simulink model "TemperatureControl"  (R2023b)
settings: Solver=VariableStepAuto  StartTime=0.0  StopTime=10.0  RelTol=1e-3
model workspace (MAT data in the model file):
  COOLING = 1
  TEMPDES = 2
  agentf = 1
libraries: rllib x1
settings Model: Creator=mail  LastModifiedBy=juliu
settings DebuggingCC: UnconnectedInputMsg=warning  UnconnectedOutputMsg=warning  UnconnectedLineMsg=warning
settings ModelReferenceCC: EnableRefExpFcnMdlSchedulingChecks=on
settings RTWCC: DLArmComputeVersion=19.05

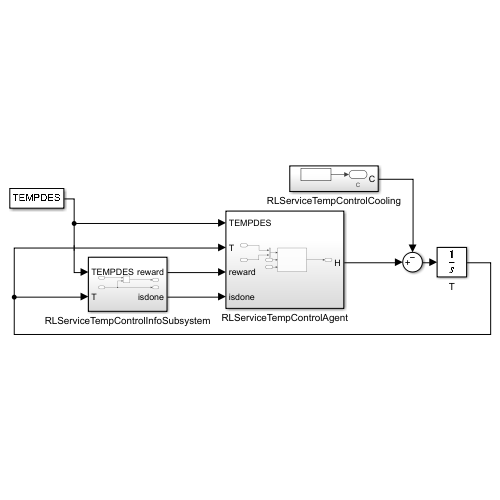
[thumbnail: Simulink's stored preview of the top-level diagram]
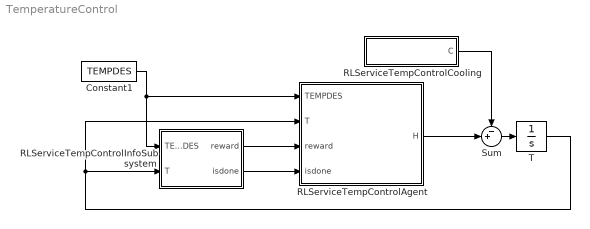
== system TemperatureControl ==
  Constant1 : Constant  Value=TEMPDES
  RLServiceTempControlAgent : Subsystem
  RLServiceTempControlCooling : Subsystem
  RLServiceTempControlInfoSubsystem : Subsystem
  Sum : Sum  Inputs=-+|
  T : Integrator
  wires:
  Sum/1 -> T/1
  T/1 -> RLServiceTempControlInfoSubsystem/2(T), RLServiceTempControlAgent/2(T)
  Constant1/1 -> RLServiceTempControlInfoSubsystem/1(TEMPDES), RLServiceTempControlAgent/1(TEMPDES)
  RLServiceTempControlInfoSubsystem/1(reward) -> RLServiceTempControlAgent/3(reward)
  RLServiceTempControlInfoSubsystem/2(isdone) -> RLServiceTempControlAgent/4(isdone)
  RLServiceTempControlAgent/1(H) -> Sum/2
  RLServiceTempControlCooling/1(C) -> Sum/1

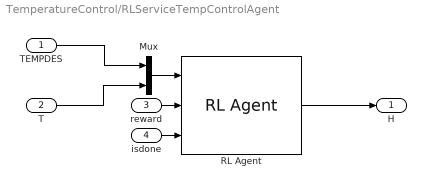
== system TemperatureControl/RLServiceTempControlAgent ==
  TEMPDES : Inport
  T : Inport  Port=2
  reward : Inport  Port=3
  isdone : Inport  Port=4
  Mux : Mux  Inputs=2
  RL Agent : rllib/RL Agent  Agent=agentf  ExternalActionAsInput=off  ProvideCumRwd=off  TreatAsDirectFeedthrough=on
  H : Outport
  wires:
  T/1 -> Mux/2
  isdone/1 -> RL Agent/3
  reward/1 -> RL Agent/2
  RL Agent/1 -> H/1
  TEMPDES/1 -> Mux/1
  Mux/1 -> RL Agent/1

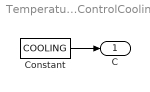
== system TemperatureControl/RLServiceTempControlCooling ==
  Constant : Constant  Value=COOLING
  C : Outport
  wires:
  Constant/1 -> C/1

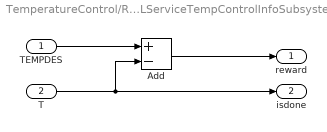
== system TemperatureControl/RLServiceTempControlInfoSubsystem ==
  TEMPDES : Inport
  T : Inport  Port=2
  Add : Sum  Inputs=+-
  reward : Outport
  isdone : Outport  Port=2
  wires:
  T/1 -> Add/2, isdone/1
  TEMPDES/1 -> Add/1
  Add/1 -> reward/1
